simulink model "kopter_se_zavazim_LQR"  (R2024b)
settings: Solver=FixedStepAuto  StartTime=0.0  StopTime=30  FixedStep=0.01  RelTol=1e-3
values from neighbouring files (symbols this model uses):
  b_moment = 5.4e-6    (= 5.4e-06)    [parametry_kopter_se_zavazim.m]
  d = 1    [parametry_kopter_se_zavazim.m]
  g = 9.81    [parametry_kopter_se_zavazim.m]
  Ip = m*d^2    (= 1)    [parametry_kopter_se_zavazim.m]
  Ixx = 0.0222    [parametry_kopter_se_zavazim.m]
  Iyy = 0.0222    [parametry_kopter_se_zavazim.m]
  Izz = 0.0429    [parametry_kopter_se_zavazim.m]
  k_thrust = 2.3e-3    (= 0.0023)    [parametry_kopter_se_zavazim.m]
  ki_lqr = K_ex_lqr(:, 17:20)    [odvozeni_stavova_regulace_OTHER_ANGLES.m]
  kimot_lqr = Kmot_ex_lqr(:, 17:20)    [odvozeni_stavova_regulace_OTHER_ANGLES.m]
  kp_lqr = K_ex_lqr(:, 1:16)    [odvozeni_stavova_regulace_OTHER_ANGLES.m]
  kpmot_lqr = Kmot_ex_lqr(:, 1:16)    [odvozeni_stavova_regulace_OTHER_ANGLES.m]
  l = 0.2051    [parametry_kopter_se_zavazim.m]
  L_observer = place(Ac', Cc', poles_obs)'    [odvozeni_stavova_regulace_OTHER_ANGLES.m]
  M = 2    [parametry_kopter_se_zavazim.m]
  m = 1    [parametry_kopter_se_zavazim.m]
  Us_p = [(M+m)*g; 0; 0; 0]    [parametry_kopter_se_zavazim.m]
  Xinit_ss = [Xinit_matrix; [0 0 0 0 0 0 0 0]']    [parametry_kopter_se_zavazim.m]
  Xs_p = [0;0;0; 0;0;0; 0;0; 0;0;0; 0;0;0; 0;0]    [parametry_kopter_se_zavazim.m]
undefined symbols (not defined in the file or in its folder): L
libraries: simulink_extras x10
(part 2 of 3)

== matlab function kopter_se_zavazim_LQR/Nelinearni State-Space (se zavazim)_other_angles_motors/Bm ==
  data: roll input; Bm output; pitch input; yaw input; alpha input; beta input; M parameter; Ixx parameter; Iyy parameter; Izz parameter; d parameter; m parameter; k_thrust parameter; b_moment parameter; l parameter
function Bm = fcn(roll, pitch, yaw, alpha, beta, M, Ixx, Iyy, Izz, d, m, k_thrust, b_moment, l)
% Matice vstupu do soustavy kvadrokoptery se zavazim

phi_t = roll;
theta_t = pitch;
psi_t = yaw;

alpha_t = alpha;
beta_t = beta;

Bm = [ 
                                                                                                                                                                                                                                                                                                                                                                                                                                                                                                                                                                                              0,                                                                                                                                                                                                                                                                                                                                                                                                                                                                                                                                                                                               0,                                                                                                                                                                                                                                                                                                                                                                                                                                                                                                                                                                                               0,                                                                                                                                                                                                                                                                                                                                                                                                                                                                                                                                                                                               0;
                                                                                                                                                                                                                                                                                                                                                                                                                                                                                                                                                                                              0,                                                                                                                                                                                                                                                                                                                                                                                                                                                                                                                                                                                               0,                                                                                                                                                                                                                                                                                                                                                                                                                                                                                                                                                                                               0,                                                                                                                                                                                                                                                                                                                                                                                                                                                                                                                                                                                               0;
                                                                                                                                                                                                                                                                                                                                                                                                                                                                                                                                                                                              0,                                                                                                                                                                                                                                                                                                                                                                                                                                                                                                                                                                                               0,                                                                                                                                                                                                                                                                                                                                                                                                                                                                                                                                                                                               0,                                                                                                                                                                                                                                                                                                                                                                                                                                                                                                                                                                                               0;
                                                                                                                                                                                                                                                                                                                                                                                                                                                                                                                                                                                              0,                                                                                                                                                                                                                                                                                                                                                                                                                                                                                                                                                                                               0,                                                                                                                                                                                                                                                                                                                                                                                                                                                                                                                                                                                               0,                                                                                                                                                                                                                                                                                                                                                                                                                                                                                                                                                                                               0;
                                                                                                                                                                                                                                                                                                                                                                                                                                                                                                                                                                                              0,                                                                                                                                                                                                                                                                                                                                                                                                                                                                                                                                                                                               0,                                                                                                                                                                                                                                                                                                                                                                                                                                                                                                                                                                                               0,                                                                                                                                                                                                                                                                                                                                                                                                                                                                                                                                                                                               0;
                                                                                                                                                                                                                                                                                                                                                                                                                                                                                                                                                                                              0,                                                                                                                                                                                                                                                                                                                                                                                                                                                                                                                                                                                               0,                                                                                                                                                                                                                                                                                                                                                                                                                                                                                                                                                                                               0,                                                                                                                                                                                                                                                                                                                                                                                                                                                                                                                                                                                               0;
                                                                                                                                                                                                                                                                                                                                                                                                                                                                                                                                                                                              0,                                                                                                                                                                                                                                                                                                                                                                                                                                                                                                                                                                                               0,                                                                                                                                                                                                                                                                                                                                                                                                                                                                                                                                                                                               0,                                                                                                                                                                                                                                                                                                                                                                                                                                                                                                                                                                                               0;
                                                                                                                                                                                                                                                                                                                                                                                                                                                                                                                                                                                              0,                                                                                                                                                                                                                                                                                                                                                                                                                                                                                                                                                                                               0,                                                                                                                                                                                                                                                                                                                                                                                                                                                                                                                                                                                               0,                                                                                                                                                                                                                                                                                                                                                                                                                                                                                                                                                                                               0;
(k_thrust*(M*sin(phi_t)*sin(psi_t) + m*sin(phi_t)*sin(psi_t) + M*cos(phi_t)*cos(psi_t)*sin(theta_t) + m*cos(phi_t)*cos(psi_t)*sin(theta_t) - m*cos(beta_t)^2*sin(phi_t)*sin(psi_t) - m*cos(beta_t)^2*cos(phi_t)*cos(psi_t)*sin(theta_t) + m*cos(alpha_t)^2*cos(beta_t)^2*sin(phi_t)*sin(psi_t) + m*cos(alpha_t)*cos(beta_t)^2*cos(phi_t)*sin(alpha_t)*cos(theta_t) + m*cos(alpha_t)^2*cos(beta_t)^2*cos(phi_t)*cos(psi_t)*sin(theta_t) + m*cos(beta_t)*cos(psi_t)*sin(alpha_t)*sin(beta_t)*sin(phi_t) - m*cos(beta_t)*cos(phi_t)*sin(alpha_t)*sin(beta_t)*sin(psi_t)*sin(theta_t)))/(M*(M + m)), (k_thrust*(M*sin(phi_t)*sin(psi_t) + m*sin(phi_t)*sin(psi_t) + M*cos(phi_t)*cos(psi_t)*sin(theta_t) + m*cos(phi_t)*cos(psi_t)*sin(theta_t) - m*cos(beta_t)^2*sin(phi_t)*sin(psi_t) - m*cos(beta_t)^2*cos(phi_t)*cos(psi_t)*sin(theta_t) + m*cos(alpha_t)^2*cos(beta_t)^2*sin(phi_t)*sin(psi_t) + m*cos(alpha_t)*cos(beta_t)^2*cos(phi_t)*sin(alpha_t)*cos(theta_t) + m*cos(alpha_t)^2*cos(beta_t)^2*cos(phi_t)*cos(psi_t)*sin(theta_t) + m*cos(beta_t)*cos(psi_t)*sin(alpha_t)*sin(beta_t)*sin(phi_t) - m*cos(beta_t)*cos(phi_t)*sin(alpha_t)*sin(beta_t)*sin(psi_t)*sin(theta_t)))/(M*(M + m)), (k_thrust*(M*sin(phi_t)*sin(psi_t) + m*sin(phi_t)*sin(psi_t) + M*cos(phi_t)*cos(psi_t)*sin(theta_t) + m*cos(phi_t)*cos(psi_t)*sin(theta_t) - m*cos(beta_t)^2*sin(phi_t)*sin(psi_t) - m*cos(beta_t)^2*cos(phi_t)*cos(psi_t)*sin(theta_t) + m*cos(alpha_t)^2*cos(beta_t)^2*sin(phi_t)*sin(psi_t) + m*cos(alpha_t)*cos(beta_t)^2*cos(phi_t)*sin(alpha_t)*cos(theta_t) + m*cos(alpha_t)^2*cos(beta_t)^2*cos(phi_t)*cos(psi_t)*sin(theta_t) + m*cos(beta_t)*cos(psi_t)*sin(alpha_t)*sin(beta_t)*sin(phi_t) - m*cos(beta_t)*cos(phi_t)*sin(alpha_t)*sin(beta_t)*sin(psi_t)*sin(theta_t)))/(M*(M + m)), (k_thrust*(M*sin(phi_t)*sin(psi_t) + m*sin(phi_t)*sin(psi_t) + M*cos(phi_t)*cos(psi_t)*sin(theta_t) + m*cos(phi_t)*cos(psi_t)*sin(theta_t) - m*cos(beta_t)^2*sin(phi_t)*sin(psi_t) - m*cos(beta_t)^2*cos(phi_t)*cos(psi_t)*sin(theta_t) + m*cos(alpha_t)^2*cos(beta_t)^2*sin(phi_t)*sin(psi_t) + m*cos(alpha_t)*cos(beta_t)^2*cos(phi_t)*sin(alpha_t)*cos(theta_t) + m*cos(alpha_t)^2*cos(beta_t)^2*cos(phi_t)*cos(psi_t)*sin(theta_t) + m*cos(beta_t)*cos(psi_t)*sin(alpha_t)*sin(beta_t)*sin(phi_t) - m*cos(beta_t)*cos(phi_t)*sin(alpha_t)*sin(beta_t)*sin(psi_t)*sin(theta_t)))/(M*(M + m));
                                                                                                                                                                                              -(k_thrust*(M*cos(psi_t)*sin(phi_t) - M*cos(phi_t)*sin(psi_t)*sin(theta_t) + m*cos(beta_t)^2*cos(psi_t)*sin(phi_t) - m*cos(beta_t)^2*cos(phi_t)*sin(psi_t)*sin(theta_t) + m*cos(beta_t)*sin(alpha_t)*sin(beta_t)*sin(phi_t)*sin(psi_t) - m*cos(alpha_t)*cos(beta_t)*cos(phi_t)*sin(beta_t)*cos(theta_t) + m*cos(beta_t)*cos(phi_t)*cos(psi_t)*sin(alpha_t)*sin(beta_t)*sin(theta_t)))/(M*(M + m)),                                                                                                                                                                                               -(k_thrust*(M*cos(psi_t)*sin(phi_t) - M*cos(phi_t)*sin(psi_t)*sin(theta_t) + m*cos(beta_t)^2*cos(psi_t)*sin(phi_t) - m*cos(beta_t)^2*cos(phi_t)*sin(psi_t)*sin(theta_t) + m*cos(beta_t)*sin(alpha_t)*sin(beta_t)*sin(phi_t)*sin(psi_t) - m*cos(alpha_t)*cos(beta_t)*cos(phi_t)*sin(beta_t)*cos(theta_t) + m*cos(beta_t)*cos(phi_t)*cos(psi_t)*sin(alpha_t)*sin(beta_t)*sin(theta_t)))/(M*(M + m)),                                                                                                                                                                                               -(k_thrust*(M*cos(psi_t)*sin(phi_t) - M*cos(phi_t)*sin(psi_t)*sin(theta_t) + m*cos(beta_t)^2*cos(psi_t)*sin(phi_t) - m*cos(beta_t)^2*cos(phi_t)*sin(psi_t)*sin(theta_t) + m*cos(beta_t)*sin(alpha_t)*sin(beta_t)*sin(phi_t)*sin(psi_t) - m*cos(alpha_t)*cos(beta_t)*cos(phi_t)*sin(beta_t)*cos(theta_t) + m*cos(beta_t)*cos(phi_t)*cos(psi_t)*sin(alpha_t)*sin(beta_t)*sin(theta_t)))/(M*(M + m)),                                                                                                                                                                                               -(k_thrust*(M*cos(psi_t)*sin(phi_t) - M*cos(phi_t)*sin(psi_t)*sin(theta_t) + m*cos(beta_t)^2*cos(psi_t)*sin(phi_t) - m*cos(beta_t)^2*cos(phi_t)*sin(psi_t)*sin(theta_t) + m*cos(beta_t)*sin(alpha_t)*sin(beta_t)*sin(phi_t)*sin(psi_t) - m*cos(alpha_t)*cos(beta_t)*cos(phi_t)*sin(beta_t)*cos(theta_t) + m*cos(beta_t)*cos(phi_t)*cos(psi_t)*sin(alpha_t)*sin(beta_t)*sin(theta_t)))/(M*(M + m));
                                                                                                                                                            (k_thrust*(M*cos(phi_t)*cos(theta_t) + m*cos(phi_t)*cos(theta_t) - m*cos(alpha_t)^2*cos(beta_t)^2*cos(phi_t)*cos(theta_t) + m*cos(alpha_t)*cos(beta_t)^2*sin(alpha_t)*sin(phi_t)*sin(psi_t) - m*cos(alpha_t)*cos(beta_t)*cos(psi_t)*sin(beta_t)*sin(phi_t) + m*cos(alpha_t)*cos(beta_t)^2*cos(phi_t)*cos(psi_t)*sin(alpha_t)*sin(theta_t) + m*cos(alpha_t)*cos(beta_t)*cos(phi_t)*sin(beta_t)*sin(psi_t)*sin(theta_t)))/(M*(M + m)),                                                                                                                                                             (k_thrust*(M*cos(phi_t)*cos(theta_t) + m*cos(phi_t)*cos(theta_t) - m*cos(alpha_t)^2*cos(beta_t)^2*cos(phi_t)*cos(theta_t) + m*cos(alpha_t)*cos(beta_t)^2*sin(alpha_t)*sin(phi_t)*sin(psi_t) - m*cos(alpha_t)*cos(beta_t)*cos(psi_t)*sin(beta_t)*sin(phi_t) + m*cos(alpha_t)*cos(beta_t)^2*cos(phi_t)*cos(psi_t)*sin(alpha_t)*sin(theta_t) + m*cos(alpha_t)*cos(beta_t)*cos(phi_t)*sin(beta_t)*sin(psi_t)*sin(theta_t)))/(M*(M + m)),                                                                                                                                                             (k_thrust*(M*cos(phi_t)*cos(theta_t) + m*cos(phi_t)*cos(theta_t) - m*cos(alpha_t)^2*cos(beta_t)^2*cos(phi_t)*cos(theta_t) + m*cos(alpha_t)*cos(beta_t)^2*sin(alpha_t)*sin(phi_t)*sin(psi_t) - m*cos(alpha_t)*cos(beta_t)*cos(psi_t)*sin(beta_t)*sin(phi_t) + m*cos(alpha_t)*cos(beta_t)^2*cos(phi_t)*cos(psi_t)*sin(alpha_t)*sin(theta_t) + m*cos(alpha_t)*cos(beta_t)*cos(phi_t)*sin(beta_t)*sin(psi_t)*sin(theta_t)))/(M*(M + m)),                                                                                                                                                             (k_thrust*(M*cos(phi_t)*cos(theta_t) + m*cos(phi_t)*cos(theta_t) - m*cos(alpha_t)^2*cos(beta_t)^2*cos(phi_t)*cos(theta_t) + m*cos(alpha_t)*cos(beta_t)^2*sin(alpha_t)*sin(phi_t)*sin(psi_t) - m*cos(alpha_t)*cos(beta_t)*cos(psi_t)*sin(beta_t)*sin(phi_t) + m*cos(alpha_t)*cos(beta_t)^2*cos(phi_t)*cos(psi_t)*sin(alpha_t)*sin(theta_t) + m*cos(alpha_t)*cos(beta_t)*cos(phi_t)*sin(beta_t)*sin(psi_t)*sin(theta_t)))/(M*(M + m));
                            (Ixx*Izz*b_moment*sin(theta_t) + Ixx*Izz*k_thrust*l - Ixx*Izz*k_thrust*l*cos(theta_t)^2 + Iyy*Izz*k_thrust*l*cos(theta_t)^2 + Ixx*Iyy*b_moment*cos(phi_t)^2*sin(theta_t) - Ixx*Izz*b_moment*cos(phi_t)^2*sin(theta_t) + Ixx*Iyy*k_thrust*l*cos(phi_t)^2 - Ixx*Izz*k_thrust*l*cos(phi_t)^2 - Ixx*Iyy*k_thrust*l*cos(phi_t)^2*cos(theta_t)^2 + Ixx*Izz*k_thrust*l*cos(phi_t)^2*cos(theta_t)^2 + Ixx*Iyy*k_thrust*l*cos(phi_t)*cos(theta_t)*sin(phi_t)*sin(theta_t) - Ixx*Izz*k_thrust*l*cos(phi_t)*cos(theta_t)*sin(phi_t)*sin(theta_t))/(Ixx*Iyy*Izz*cos(theta_t)^2),                            -(Ixx*Izz*b_moment*sin(theta_t) + Ixx*Izz*k_thrust*l - Ixx*Izz*k_thrust*l*cos(theta_t)^2 + Iyy*Izz*k_thrust*l*cos(theta_t)^2 + Ixx*Iyy*b_moment*cos(phi_t)^2*sin(theta_t) - Ixx*Izz*b_moment*cos(phi_t)^2*sin(theta_t) + Ixx*Iyy*k_thrust*l*cos(phi_t)^2 - Ixx*Izz*k_thrust*l*cos(phi_t)^2 - Ixx*Iyy*k_thrust*l*cos(phi_t)^2*cos(theta_t)^2 + Ixx*Izz*k_thrust*l*cos(phi_t)^2*cos(theta_t)^2 - Ixx*Iyy*k_thrust*l*cos(phi_t)*cos(theta_t)*sin(phi_t)*sin(theta_t) + Ixx*Izz*k_thrust*l*cos(phi_t)*cos(theta_t)*sin(phi_t)*sin(theta_t))/(Ixx*Iyy*Izz*cos(theta_t)^2),                             (Ixx*Izz*b_moment*sin(theta_t) - Ixx*Izz*k_thrust*l + Ixx*Izz*k_thrust*l*cos(theta_t)^2 - Iyy*Izz*k_thrust*l*cos(theta_t)^2 + Ixx*Iyy*b_moment*cos(phi_t)^2*sin(theta_t) - Ixx*Izz*b_moment*cos(phi_t)^2*sin(theta_t) - Ixx*Iyy*k_thrust*l*cos(phi_t)^2 + Ixx*Izz*k_thrust*l*cos(phi_t)^2 + Ixx*Iyy*k_thrust*l*cos(phi_t)^2*cos(theta_t)^2 - Ixx*Izz*k_thrust*l*cos(phi_t)^2*cos(theta_t)^2 - Ixx*Iyy*k_thrust*l*cos(phi_t)*cos(theta_t)*sin(phi_t)*sin(theta_t) + Ixx*Izz*k_thrust*l*cos(phi_t)*cos(theta_t)*sin(phi_t)*sin(theta_t))/(Ixx*Iyy*Izz*cos(theta_t)^2),                            -(Ixx*Izz*b_moment*sin(theta_t) - Ixx*Izz*k_thrust*l + Ixx*Izz*k_thrust*l*cos(theta_t)^2 - Iyy*Izz*k_thrust*l*cos(theta_t)^2 + Ixx*Iyy*b_moment*cos(phi_t)^2*sin(theta_t) - Ixx*Izz*b_moment*cos(phi_t)^2*sin(theta_t) - Ixx*Iyy*k_thrust*l*cos(phi_t)^2 + Ixx*Izz*k_thrust*l*cos(phi_t)^2 + Ixx*Iyy*k_thrust*l*cos(phi_t)^2*cos(theta_t)^2 - Ixx*Izz*k_thrust*l*cos(phi_t)^2*cos(theta_t)^2 + Ixx*Iyy*k_thrust*l*cos(phi_t)*cos(theta_t)*sin(phi_t)*sin(theta_t) - Ixx*Izz*k_thrust*l*cos(phi_t)*cos(theta_t)*sin(phi_t)*sin(theta_t))/(Ixx*Iyy*Izz*cos(theta_t)^2);
                                                                                                                                                                                                                                                                                                                                                                  -(Iyy*b_moment*sin(2*phi_t) - Izz*b_moment*sin(2*phi_t) + Iyy*k_thrust*l*cos(theta_t) + Izz*k_thrust*l*cos(theta_t) - Iyy*k_thrust*l*cos(2*phi_t + theta_t) + Izz*k_thrust*l*cos(2*phi_t + theta_t))/(2*Iyy*Izz*cos(theta_t)),                                                                                                                                                                                                                                                                                                                                                                   -(Izz*b_moment*sin(2*phi_t) - Iyy*b_moment*sin(2*phi_t) + Iyy*k_thrust*l*cos(theta_t) + Izz*k_thrust*l*cos(theta_t) - Iyy*k_thrust*l*cos(2*phi_t - theta_t) + Izz*k_thrust*l*cos(2*phi_t - theta_t))/(2*Iyy*Izz*cos(theta_t)),                                                                                                                                                                                                                                                                                                                                                                    (Izz*b_moment*sin(2*phi_t) - Iyy*b_moment*sin(2*phi_t) + Iyy*k_thrust*l*cos(theta_t) + Izz*k_thrust*l*cos(theta_t) - Iyy*k_thrust*l*cos(2*phi_t + theta_t) + Izz*k_thrust*l*cos(2*phi_t + theta_t))/(2*Iyy*Izz*cos(theta_t)),                                                                                                                                                                                                                                                                                                                                                                    (Iyy*b_moment*sin(2*phi_t) - Izz*b_moment*sin(2*phi_t) + Iyy*k_thrust*l*cos(theta_t) + Izz*k_thrust*l*cos(theta_t) - Iyy*k_thrust*l*cos(2*phi_t - theta_t) + Izz*k_thrust*l*cos(2*phi_t - theta_t))/(2*Iyy*Izz*cos(theta_t));
                                                                                                                                                                                                                                                                                                                                   (Iyy*b_moment + Izz*b_moment + Iyy*b_moment*cos(2*phi_t) - Izz*b_moment*cos(2*phi_t) + Iyy*k_thrust*l*sin(theta_t) + Izz*k_thrust*l*sin(theta_t) + Iyy*k_thrust*l*sin(2*phi_t + theta_t) - Izz*k_thrust*l*sin(2*phi_t + theta_t))/(2*Iyy*Izz*cos(theta_t)^2),                                                                                                                                                                                                                                                                                                                                   -(Iyy*b_moment + Izz*b_moment + Iyy*b_moment*cos(2*phi_t) - Izz*b_moment*cos(2*phi_t) + Iyy*k_thrust*l*sin(theta_t) + Izz*k_thrust*l*sin(theta_t) - Iyy*k_thrust*l*sin(2*phi_t - theta_t) + Izz*k_thrust*l*sin(2*phi_t - theta_t))/(2*Iyy*Izz*cos(theta_t)^2),                                                                                                                                                                                                                                                                                                                                    (Iyy*b_moment + Izz*b_moment + Iyy*b_moment*cos(2*phi_t) - Izz*b_moment*cos(2*phi_t) - Iyy*k_thrust*l*sin(theta_t) - Izz*k_thrust*l*sin(theta_t) - Iyy*k_thrust*l*sin(2*phi_t + theta_t) + Izz*k_thrust*l*sin(2*phi_t + theta_t))/(2*Iyy*Izz*cos(theta_t)^2),                                                                                                                                                                                                                                                                                                                                   -(Iyy*b_moment + Izz*b_moment + Iyy*b_moment*cos(2*phi_t) - Izz*b_moment*cos(2*phi_t) - Iyy*k_thrust*l*sin(theta_t) - Izz*k_thrust*l*sin(theta_t) + Iyy*k_thrust*l*sin(2*phi_t - theta_t) - Izz*k_thrust*l*sin(2*phi_t - theta_t))/(2*Iyy*Izz*cos(theta_t)^2);
                                                                                                                                                                                                                                                                                                                                                                                                                                    -(k_thrust*(cos(phi_t)*sin(alpha_t)*cos(theta_t) + cos(alpha_t)*sin(phi_t)*sin(psi_t) + cos(alpha_t)*cos(phi_t)*cos(psi_t)*sin(theta_t)))/(M*d*cos(beta_t)),                                                                                                                                                                                                                                                                                                                                                                                                                                     -(k_thrust*(cos(phi_t)*sin(alpha_t)*cos(theta_t) + cos(alpha_t)*sin(phi_t)*sin(psi_t) + cos(alpha_t)*cos(phi_t)*cos(psi_t)*sin(theta_t)))/(M*d*cos(beta_t)),                                                                                                                                                                                                                                                                                                                                                                                                                                     -(k_thrust*(cos(phi_t)*sin(alpha_t)*cos(theta_t) + cos(alpha_t)*sin(phi_t)*sin(psi_t) + cos(alpha_t)*cos(phi_t)*cos(psi_t)*sin(theta_t)))/(M*d*cos(beta_t)),                                                                                                                                                                                                                                                                                                                                                                                                                                     -(k_thrust*(cos(phi_t)*sin(alpha_t)*cos(theta_t) + cos(alpha_t)*sin(phi_t)*sin(psi_t) + cos(alpha_t)*cos(phi_t)*cos(psi_t)*sin(theta_t)))/(M*d*cos(beta_t));
                                                                                                                                                                                                                                                                                                                        (k_thrust*(cos(beta_t)*cos(psi_t)*sin(phi_t) - cos(alpha_t)*cos(phi_t)*sin(beta_t)*cos(theta_t) - cos(beta_t)*cos(phi_t)*sin(psi_t)*sin(theta_t) + sin(alpha_t)*sin(beta_t)*sin(phi_t)*sin(psi_t) + cos(phi_t)*cos(psi_t)*sin(alpha_t)*sin(beta_t)*sin(theta_t)))/(M*d),                                                                                                                                                                                                                                                                                                                         (k_thrust*(cos(beta_t)*cos(psi_t)*sin(phi_t) - cos(alpha_t)*cos(phi_t)*sin(beta_t)*cos(theta_t) - cos(beta_t)*cos(phi_t)*sin(psi_t)*sin(theta_t) + sin(alpha_t)*sin(beta_t)*sin(phi_t)*sin(psi_t) + cos(phi_t)*cos(psi_t)*sin(alpha_t)*sin(beta_t)*sin(theta_t)))/(M*d),                                                                                                                                                                                                                                                                                                                         (k_thrust*(cos(beta_t)*cos(psi_t)*sin(phi_t) - cos(alpha_t)*cos(phi_t)*sin(beta_t)*cos(theta_t) - cos(beta_t)*cos(phi_t)*sin(psi_t)*sin(theta_t) + sin(alpha_t)*sin(beta_t)*sin(phi_t)*sin(psi_t) + cos(phi_t)*cos(psi_t)*sin(alpha_t)*sin(beta_t)*sin(theta_t)))/(M*d),                                                                                                                                                                                                                                                                                                                         (k_thrust*(cos(beta_t)*cos(psi_t)*sin(phi_t) - cos(alpha_t)*cos(phi_t)*sin(beta_t)*cos(theta_t) - cos(beta_t)*cos(phi_t)*sin(psi_t)*sin(theta_t) + sin(alpha_t)*sin(beta_t)*sin(phi_t)*sin(psi_t) + cos(phi_t)*cos(psi_t)*sin(alpha_t)*sin(beta_t)*sin(theta_t)))/(M*d)];

== matlab function kopter_se_zavazim_LQR/Nelinearni State-Space (se zavazim)_other_angles_motors/BQ ==
  data: BQ output; g parameter
function BQ = fcn(g)
% Matice vstupu tihy
BQ = [0 0 0 0 0 0 0 0 0 0 -g 0 0 0 0 0]';

== matlab function kopter_se_zavazim_LQR/otacky^2 na sily ==
  data: U input; Forces output; l parameter; b_moment parameter; k_thrust parameter
function Forces = fcn(U, l, b_moment, k_thrust)
U1 = U(1);
U2 = U(2);
U3 = U(3);
U4 = U(4);

T = k_thrust*(U1 + U2 + U3 + U4);
Tau_phi = k_thrust*l*(U1 - U2 - U3 + U4);
Tau_theta = -k_thrust*l*(U1 + U2 - U3 - U4);
Tau_psi = b_moment*(U1 - U2 + U3 - U4);

Forces = [T; Tau_phi; Tau_theta; Tau_psi];
